simulink model "MA_Diaphragm_3DOF_linear"  (R2021b)
settings: Solver=VariableStepAuto  StartTime=0.0  StopTime=0.5  RelTol=1e-3
undefined symbols (not defined in the file): ma, me
libraries: fl_lib x16, acoustical_lib x8, nesl_utility x4
settings Model: Creator=김웅지  LastModifiedBy=김웅지

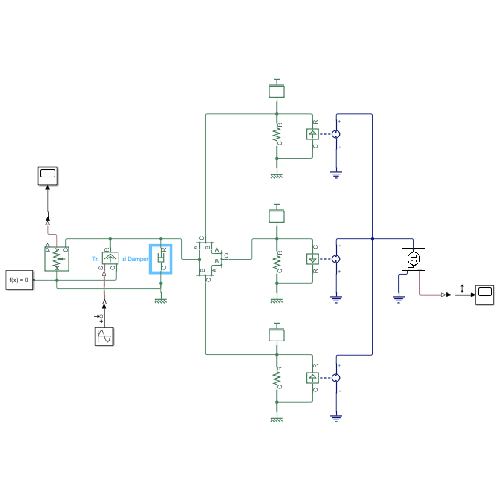
[thumbnail: Simulink's stored preview of the top-level diagram]
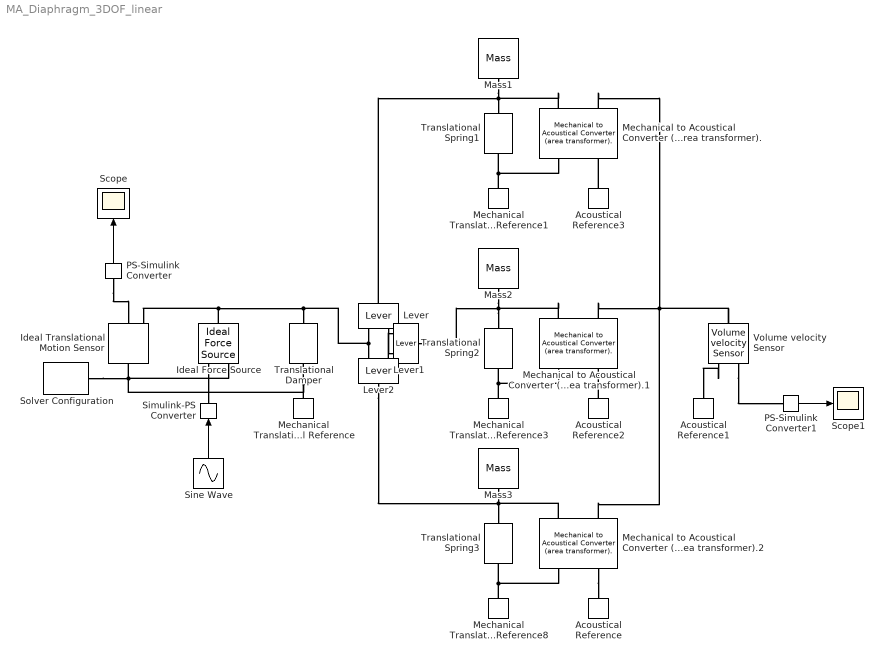
== system MA_Diaphragm_3DOF_linear ==
  Acoustical Reference{,1..3} (4 alike) : acoustical_lib/Acoustical Elements/Acoustical Reference
      settings: SourceProductName=Acoustical  InternalSimscapePortConfiguration="{\"Bottom\":[],\"Left\":[{\"id\":\"pp\",\"label\":\"\",\"type\":\"acoustical.acoustical\"}],\"Right\":[],\"Top\":[]}"
  Ideal Force Source : fl_lib/Mechanical/Mechanical Sources/Ideal Force Source
  Ideal Translational Motion Sensor : fl_lib/Mechanical/Mechanical Sensors/Ideal Translational Motion Sensor  offset=0 m
  Lever : fl_lib/Mechanical/Mechanisms/Lever  arm_AC=0.1 m  arm_BC=0.1 m  f_A_specify=off  f_A_priority=None  f_A=0 N  f_A_nominal_specify=off  f_A_nominal_unit=N  f_A_nominal_value=1  f_B_specify=off  f_B_priority=None  f_B=0 N  f_B_nominal_specify=off  f_B_nominal_unit=N  f_B_nominal_value=1  f_C_specify=off  f_C_priority=None  f_C=0 N  f_C_nominal_specify=off  f_C_nominal_unit=N  f_C_nominal_value=1
      settings: SourceProductBaseCode=SS  InternalSimscapePortConfiguration="{\"Bottom\":[],\"Left\":[{\"id\":\"A\",\"label\":\"A\",\"type\":\"foundation.mechanical.translational.translational\"},{\"id\":\"B\",\"label\":\"B\",\"type\":\"foundation.mechanical.translational.translational\"}],\"Right\":[{\"id\":\"C\",\"label\":\"C\",\"type\":\"foundation.mechanical.translational.translational\"}],\"Top\":[]}"
  Lever1 : fl_lib/Mechanical/Mechanisms/Lever  arm_AC=0.1 m  arm_BC=0.1 m  f_A_specify=off  f_A_priority=None  f_A=0 N  f_A_nominal_specify=off  f_A_nominal_unit=N  f_A_nominal_value=1  f_B_specify=off  f_B_priority=None  f_B=0 N  f_B_nominal_specify=off  f_B_nominal_unit=N  f_B_nominal_value=1  f_C_specify=off  f_C_priority=None  f_C=0 N  f_C_nominal_specify=off  f_C_nominal_unit=N  f_C_nominal_value=1
      settings: SourceProductBaseCode=SS  InternalSimscapePortConfiguration="{\"Bottom\":[],\"Left\":[{\"id\":\"A\",\"label\":\"A\",\"type\":\"foundation.mechanical.translational.translational\"},{\"id\":\"B\",\"label\":\"B\",\"type\":\"foundation.mechanical.translational.translational\"}],\"Right\":[{\"id\":\"C\",\"label\":\"C\",\"type\":\"foundation.mechanical.translational.translational\"}],\"Top\":[]}"
  Lever2 : fl_lib/Mechanical/Mechanisms/Lever  arm_AC=0.1 m  arm_BC=0.1 m  f_A_specify=off  f_A_priority=None  f_A=0 N  f_A_nominal_specify=off  f_A_nominal_unit=N  f_A_nominal_value=1  f_B_specify=off  f_B_priority=None  f_B=0 N  f_B_nominal_specify=off  f_B_nominal_unit=N  f_B_nominal_value=1  f_C_specify=off  f_C_priority=None  f_C=0 N  f_C_nominal_specify=off  f_C_nominal_unit=N  f_C_nominal_value=1
      settings: SourceProductBaseCode=SS  InternalSimscapePortConfiguration="{\"Bottom\":[],\"Left\":[{\"id\":\"A\",\"label\":\"A\",\"type\":\"foundation.mechanical.translational.translational\"},{\"id\":\"B\",\"label\":\"B\",\"type\":\"foundation.mechanical.translational.translational\"}],\"Right\":[{\"id\":\"C\",\"label\":\"C\",\"type\":\"foundation.mechanical.translational.translational\"}],\"Top\":[]}"
  Mass1 : fl_lib/Mechanical/Translational Elements/Mass  mass=1/me.dl.phi(1) kg  num_ports=foundation.enum.numPorts2.one  v_specify=off  v_priority=High  v=0 m/s  v_nominal_specify=off  v_nominal_unit=m/s  v_nominal_value=1  f_specify=off  f_priority=None  f=0 N  f_nominal_specify=off  f_nominal_unit=N  f_nominal_value=1
  Mass2 : fl_lib/Mechanical/Translational Elements/Mass  mass=1/me.dl.phi(2) kg  num_ports=foundation.enum.numPorts2.one  v_specify=off  v_priority=High  v=0 m/s  v_nominal_specify=off  v_nominal_unit=m/s  v_nominal_value=1  f_specify=off  f_priority=None  f=0 N  f_nominal_specify=off  f_nominal_unit=N  f_nominal_value=1
  Mass3 : fl_lib/Mechanical/Translational Elements/Mass  mass=1/me.dl.phi(3) kg  num_ports=foundation.enum.numPorts2.one  v_specify=off  v_priority=High  v=0 m/s  v_nominal_specify=off  v_nominal_unit=m/s  v_nominal_value=1  f_specify=off  f_priority=None  f=0 N  f_nominal_specify=off  f_nominal_unit=N  f_nominal_value=1
  Mechanical Translational Reference{,1,3,8} (4 alike) : fl_lib/Mechanical/Translational Elements/Mechanical Translational Reference
  Mechanical to Acoustical Converter (area transformer). : acoustical_lib/Acoustical Elements/Mechanical to Acoustical Converter (area transformer).  Sd=ma.di.s*ma.di.psi(1) m^2  u_specify=off  u_priority=None  u=0 m^3/s  u_nominal_specify=off  u_nominal_unit=m^3/s  u_nominal_value=1  p_specify=off  p_priority=None  p=0 Pa  p_nominal_specify=off  p_nominal_unit=Pa  p_nominal_value=1  f_specify=off  f_priority=None  f=0 N  f_nominal_specify=off  f_nominal_unit=N  f_nominal_value=1  v_specify=off  v_priority=None  v=0 m/s  v_nominal_specify=off  v_nominal_unit=m/s  v_nominal_value=1
      settings: SourceProductName=Acoustical  InternalSimscapePortConfiguration="{\"Bottom\":[],\"Left\":[{\"id\":\"pp\",\"label\":\"+\",\"type\":\"acoustical.acoustical\"},{\"id\":\"R\",\"label\":\"R\",\"type\":\"foundation.mechanical.translational.translational\"}],\"Right\":[{\"id\":\"nn\",\"label\":\"-\",\"type\":\"acoustical.acoustical\"},{\"id\":\"C\",\"label\":\"C\",\"type\":\"foundation.mechanical.translational.translational\"}],\"Top\":[]}"
  Mechanical to Acoustical Converter (area transformer).1 : acoustical_lib/Acoustical Elements/Mechanical to Acoustical Converter (area transformer).  Sd=ma.di.s*ma.di.psi(2) m^2  u_specify=off  u_priority=None  u=0 m^3/s  u_nominal_specify=off  u_nominal_unit=m^3/s  u_nominal_value=1  p_specify=off  p_priority=None  p=0 Pa  p_nominal_specify=off  p_nominal_unit=Pa  p_nominal_value=1  f_specify=off  f_priority=None  f=0 N  f_nominal_specify=off  f_nominal_unit=N  f_nominal_value=1  v_specify=off  v_priority=None  v=0 m/s  v_nominal_specify=off  v_nominal_unit=m/s  v_nominal_value=1
      settings: SourceProductName=Acoustical  InternalSimscapePortConfiguration="{\"Bottom\":[],\"Left\":[{\"id\":\"pp\",\"label\":\"+\",\"type\":\"acoustical.acoustical\"},{\"id\":\"R\",\"label\":\"R\",\"type\":\"foundation.mechanical.translational.translational\"}],\"Right\":[{\"id\":\"nn\",\"label\":\"-\",\"type\":\"acoustical.acoustical\"},{\"id\":\"C\",\"label\":\"C\",\"type\":\"foundation.mechanical.translational.translational\"}],\"Top\":[]}"
  Mechanical to Acoustical Converter (area transformer).2 : acoustical_lib/Acoustical Elements/Mechanical to Acoustical Converter (area transformer).  Sd=ma.di.s*ma.di.psi(3) m^2  u_specify=off  u_priority=None  u=0 m^3/s  u_nominal_specify=off  u_nominal_unit=m^3/s  u_nominal_value=1  p_specify=off  p_priority=None  p=0 Pa  p_nominal_specify=off  p_nominal_unit=Pa  p_nominal_value=1  f_specify=off  f_priority=None  f=0 N  f_nominal_specify=off  f_nominal_unit=N  f_nominal_value=1  v_specify=off  v_priority=None  v=0 m/s  v_nominal_specify=off  v_nominal_unit=m/s  v_nominal_value=1
      settings: SourceProductName=Acoustical  InternalSimscapePortConfiguration="{\"Bottom\":[],\"Left\":[{\"id\":\"pp\",\"label\":\"+\",\"type\":\"acoustical.acoustical\"},{\"id\":\"R\",\"label\":\"R\",\"type\":\"foundation.mechanical.translational.translational\"}],\"Right\":[{\"id\":\"nn\",\"label\":\"-\",\"type\":\"acoustical.acoustical\"},{\"id\":\"C\",\"label\":\"C\",\"type\":\"foundation.mechanical.translational.translational\"}],\"Top\":[]}"
  PS-Simulink Converter : nesl_utility/PS-Simulink Converter  PhysicalDomain=network_engine_domain  SubClassName=ps_output  LeftPortType=input  RightPortType=output  PseudoPeriodic=off  Frequencies=[]  Unit=inherit  AffineConversion=off
      settings: SourceProductBaseCode=PW,SS
  PS-Simulink Converter1 : nesl_utility/PS-Simulink Converter  PhysicalDomain=network_engine_domain  SubClassName=ps_output  LeftPortType=input  RightPortType=output  PseudoPeriodic=off  Frequencies=[]  Unit=inherit  AffineConversion=off
      settings: SourceProductBaseCode=PW,SS
  Scope : Scope
  Scope1 : Scope
  Simulink-PS Converter : nesl_utility/Simulink-PS Converter  PhysicalDomain=network_engine_domain  SubClassName=ps_input  LeftPortType=input  RightPortType=output  PseudoPeriodic=off  Frequencies=[]  NoiseDistribution=none  NoiseParameters=[]  Unit=1  AffineConversion=off  FilteringAndDerivatives=provide  SimscapeFilterOrder=1  InputFilterTimeConstant=0.001  UdotUserProvided=0
      settings: SourceProductBaseCode=PW,SS
  Sine Wave : Sin  SampleTime=0
  Solver Configuration : nesl_utility/Solver Configuration  PhysicalDomain=network_engine_domain  SubClassName=solver  LeftPortType=input  RightPortType=generic  Tones=[]  Harmonics=[]  SimulateNoise=off  Profile=off  UseLocalSampling=off  EnableSwitchedLinearOptims=on  FrequencyDomain=off  UseCCode=off  RelTol=0.001  AbsTol=1e-06  MinStep=1e-09  ToWorkspace=off  RevertToSquareIcSolve=off  NumHomotopyIterations=100  PhasorMode=off  PhasorModeNumHarmonics=1  DoDC=off  ResidualTolerance=1e-09  UseLocalSolver=off  LocalSolverChoice=NE_BACKWARD_EULER_ADVANCER  LocalSolverSampleTime=0.001  DoFixedCost=off  MaxNonlinIter=3  MaxModeIter=2  ComputeImpulses=off  ImpulseIterations=2  LinearAlgebra=auto  EquationFormulation=NE_TIME_EF  DelaysMemoryBudget=1024  AutomaticFiltering=on  FilteringTimeConstant=0.001  PartitionStorageMethod=AS_NEEDED  PartitionMemoryBudget=1024  PartitionMethod=ROBUST
      settings: SourceProductBaseCode=PW,SS
  Translational Damper : fl_lib/Mechanical/Translational Elements/Translational Damper  D=me.di.R N/(m/s)  v_specify=off  v_priority=None  v=0 m/s  v_nominal_specify=off  v_nominal_unit=m/s  v_nominal_value=1  f_specify=off  f_priority=None  f=0 N  f_nominal_specify=off  f_nominal_unit=N  f_nominal_value=1
  Translational Spring1 : fl_lib/Mechanical/Translational Elements/Translational Spring  spr_rate=(2*pi*me.dl.f(1))^2/me.dl.phi(1) N/m  v_specify=off  v_priority=None  v=0 m/s  v_nominal_specify=off  v_nominal_unit=m/s  v_nominal_value=1  f_specify=off  f_priority=None  f=0 N  f_nominal_specify=off  f_nominal_unit=N  f_nominal_value=1  x_specify=off  x_priority=High  x=0 m  x_nominal_specify=off  x_nominal_unit=m  x_nominal_value=1
  Translational Spring2 : fl_lib/Mechanical/Translational Elements/Translational Spring  spr_rate=(2*pi*me.dl.f(2))^2/me.dl.phi(2) N/m  v_specify=off  v_priority=None  v=0 m/s  v_nominal_specify=off  v_nominal_unit=m/s  v_nominal_value=1  f_specify=off  f_priority=None  f=0 N  f_nominal_specify=off  f_nominal_unit=N  f_nominal_value=1  x_specify=off  x_priority=High  x=0 m  x_nominal_specify=off  x_nominal_unit=m  x_nominal_value=1
  Translational Spring3 : fl_lib/Mechanical/Translational Elements/Translational Spring  spr_rate=(2*pi*me.dl.f(3))^2/me.dl.phi(3) N/m  v_specify=off  v_priority=None  v=0 m/s  v_nominal_specify=off  v_nominal_unit=m/s  v_nominal_value=1  f_specify=off  f_priority=None  f=0 N  f_nominal_specify=off  f_nominal_unit=N  f_nominal_value=1  x_specify=off  x_priority=High  x=0 m  x_nominal_specify=off  x_nominal_unit=m  x_nominal_value=1
  Volume velocity Sensor : acoustical_lib/Acoustical Sensors/Volume velocity Sensor
      settings: SourceProductName=Acoustical  InternalSimscapePortConfiguration="{\"Bottom\":[],\"Left\":[{\"id\":\"pp\",\"label\":\"+\",\"type\":\"acoustical.acoustical\"}],\"Right\":[{\"id\":\"u\",\"label\":\"I\",\"type\":\"output\"},{\"id\":\"nn\",\"label\":\"-\",\"type\":\"acoustical.acoustical\"}],\"Top\":[]}"
  wires:
  PS-Simulink Converter/1 -> Scope/1
  Sine Wave/1 -> Simulink-PS Converter/1
  PS-Simulink Converter1/1 -> Scope1/1
  connections:
  Lever/LConn1 -- Ideal Translational Motion Sensor/RConn1 -- Ideal Force Source/LConn1 -- Translational Damper/LConn1 -- Lever2/LConn2
  Ideal Force Source/RConn2 -- Mechanical Translational Reference/LConn1 -- Translational Damper/RConn1 -- Solver Configuration/RConn1 -- Ideal Translational Motion Sensor/LConn1
  Ideal Force Source/RConn1 -- Simulink-PS Converter/RConn1
  Translational Spring1/RConn1 -- Mechanical Translational Reference1/LConn1 -- Mechanical to Acoustical Converter (area transformer)./RConn2
  Translational Spring3/RConn1 -- Mechanical Translational Reference8/LConn1 -- Mechanical to Acoustical Converter (area transformer).2/RConn2
  Translational Spring2/RConn1 -- Mechanical Translational Reference3/LConn1 -- Mechanical to Acoustical Converter (area transformer).1/LConn2
  Mass1/LConn1 -- Lever/RConn1 -- Mechanical to Acoustical Converter (area transformer)./LConn2 -- Translational Spring1/LConn1
  Translational Spring2/LConn1 -- Lever1/RConn1 -- Mechanical to Acoustical Converter (area transformer).1/RConn2 -- Mass2/LConn1
  Lever2/RConn1 -- Mechanical to Acoustical Converter (area transformer).2/LConn2 -- Mass3/LConn1 -- Translational Spring3/LConn1
  Lever2/LConn1 -- Lever1/LConn2
  Lever/LConn2 -- Lever1/LConn1
  PS-Simulink Converter/LConn1 -- Ideal Translational Motion Sensor/RConn2
  Volume velocity Sensor/RConn1 -- PS-Simulink Converter1/LConn1
  Volume velocity Sensor/RConn2 -- Acoustical Reference1/LConn1
  Mechanical to Acoustical Converter (area transformer).2/RConn1 -- Acoustical Reference/LConn1
  Acoustical Reference2/LConn1 -- Mechanical to Acoustical Converter (area transformer).1/LConn1
  Acoustical Reference3/LConn1 -- Mechanical to Acoustical Converter (area transformer)./RConn1
  Mechanical to Acoustical Converter (area transformer).1/RConn1 -- Volume velocity Sensor/LConn1 -- Mechanical to Acoustical Converter (area transformer)./LConn1 -- Mechanical to Acoustical Converter (area transformer).2/LConn1
